simulink model "zad2_modell"  (R2023a)
settings: Solver=ode45  StartTime=0.0  StopTime=Tsim  RelTol=1e-3  EnableMultiTasking=on
values from neighbouring files (symbols this model uses):
  beta = Ks*Kg*Km/(Jl*Jh*Rm)    (= 26833.3333333)    [zad2_b.m]
  Jh = 0.0021    [zad2_a.m]    (also in zad2_b.m)
  Jl = 0.0059    [zad2_a.m]    (also in zad2_b.m)
  K = acker(A_, B_, p)    [zad2_b.m]
  Kg = 70    [zad2_a.m]    (also in zad2_b.m)
  Km = 0.00767    [zad2_a.m]    (also in zad2_b.m)
  konst = m*g*h/Jl    (= -39.9050847458)    [zad2_b.m]
  Ks = 1.61    [zad2_a.m]    (also in zad2_b.m)
  Rm = 2.6    [zad2_a.m]    (also in zad2_b.m)
settings Model: Creator=Guzda  LastModifiedBy=Enio
settings SolverCC: AlgebraicLoopSolver=TrustRegion
settings DataIOCC: LimitDataPoints=on  SaveFormat=Array  SignalLoggingSaveFormat=ModelDataLogs  ReturnWorkspaceOutputs=off
settings OptimizationCC: LifeSpan=inf
settings DebuggingCC: UnderspecifiedInitializationDetection=Classic  MergeDetectMultiDrivingBlocksExec=none  MultiTaskDSMMsg=warning  MultiTaskCondExecSysMsg=none  UnconnectedInputMsg=warning  UnconnectedOutputMsg=warning  UnconnectedLineMsg=warning  StateNameClashWarn=warning  SFUnexpectedBacktrackingDiag=warning  SFNoUnconditionalDefaultTransitionDiag=warning  SFExecutionAtInitializationDiag=none  ArithmeticOperatorsInVariantConditions=warning
settings HardwareCC: ProdBitPerPointer=32  ProdBitPerSizeT=32  ProdBitPerPtrDiffT=32  ProdLargestAtomicFloat=None  ProdIntDivRoundTo=Undefined  ProdEndianess=Unspecified  ProdWordSize=32  ProdHWDeviceType=32-bit Generic
settings ModelReferenceCC: EnableRefExpFcnMdlSchedulingChecks=on  PropagateSignalLabelsOutOfModel=off
settings SFSimCC: SimUseLocalCustomCode=off  CustomCodeUndefinedFunction=UseInterfaceOnly
settings RTWCC: RTWUseLocalCustomCode=off
settings CodeAppCC: StateflowObjectComments=on
settings GRTTargetCC: TargetLangStandard=C89/C90 (ANSI)
settings ConfigComp: CovMetricSettings=dw  CovSaveCumulativeToWorkspaceVar=on  CovSaveSingleToWorkspaceVar=on  CovExternalEMLEnable=off

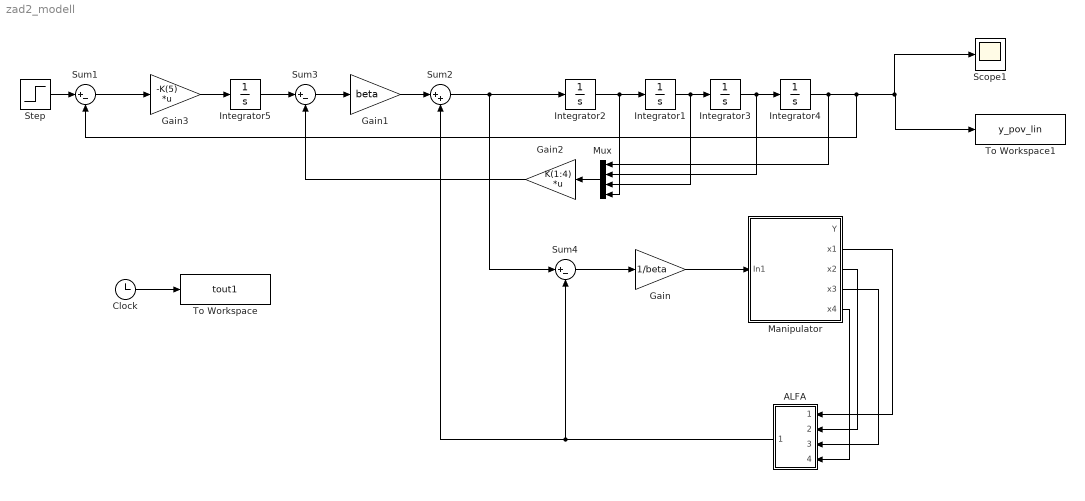
== system zad2_modell ==
  ALFA : Subsystem
  Clock : Clock
  Gain : Gain  Gain=1/beta
  Gain1 : Gain  Gain=beta
  Gain2 : Gain  Gain=K(1:4)  Multiplication=Matrix(K*u)
  Gain3 : Gain  Gain=-K(5)  Multiplication=Matrix(K*u)
  Integrator{1..5} (5 alike) : Integrator
  Manipulator : Subsystem
  Mux : Mux
  Scope1 : Scope
  Step : Step  Time=0  After=u  SampleTime=0
  Sum1 : Sum  Inputs=|+-
  Sum2 : Sum  Inputs=|++
  Sum3 : Sum  Inputs=|+-
  Sum4 : Sum  Inputs=|+-
  To Workspace : ToWorkspace  VariableName=tout1  SampleTime=-1
  To Workspace1 : ToWorkspace  VariableName=y_pov_lin  SampleTime=-1
  wires:
  Clock/1 -> To Workspace/1
  Manipulator/4(x3) -> ALFA/3(In3)
  Manipulator/5(x4) -> ALFA/4(In4)
  Manipulator/3(x2) -> ALFA/2(In2)
  Gain/1 -> Manipulator/1(In1)
  Integrator2/1 -> Mux/4, Integrator1/1
  Integrator1/1 -> Mux/3, Integrator3/1
  Integrator3/1 -> Mux/2, Integrator4/1
  Integrator4/1 -> Mux/1, Sum1/2, To Workspace1/1, Scope1/1
  ALFA/1(Out1) -> Sum4/2, Sum2/2
  Sum2/1 -> Sum4/1, Integrator2/1
  Gain1/1 -> Sum2/1
  Sum3/1 -> Gain1/1
  Mux/1 -> Gain2/1
  Gain2/1 -> Sum3/2
  Integrator5/1 -> Sum3/1
  Gain3/1 -> Integrator5/1
  Sum1/1 -> Gain3/1
  Step/1 -> Sum1/1
  Sum4/1 -> Gain/1
  Manipulator/2(x1) -> ALFA/1(In1)

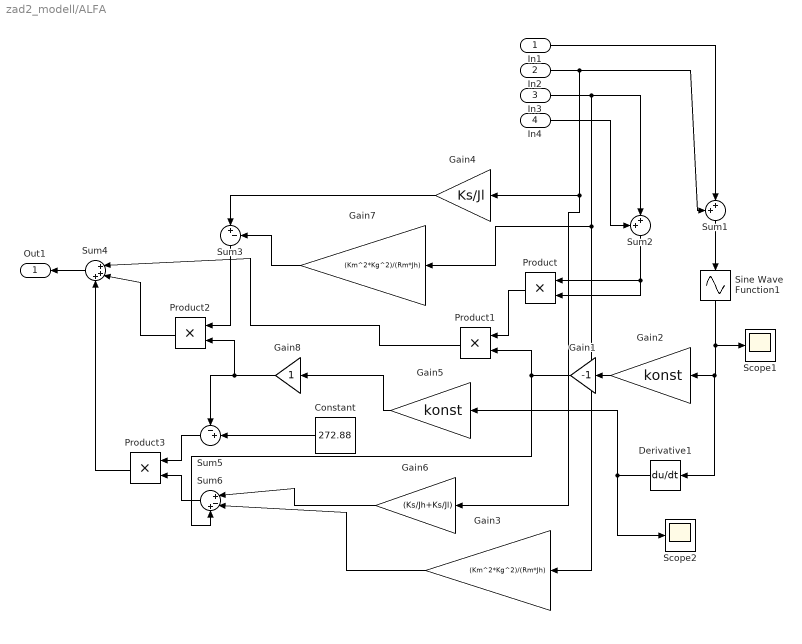
== system zad2_modell/ALFA ==
  In1 : Inport
  In2 : Inport  Port=2
  In3 : Inport  Port=3
  In4 : Inport  Port=4
  Constant : Constant  Value=272.88
  Derivative1 : Derivative
  Gain1 : Gain  Gain=-1
  Gain2 : Gain  Gain=konst
  Gain3 : Gain  Gain=(Km^2*Kg^2)/(Rm*Jh)
  Gain4 : Gain  Gain=Ks/Jl
  Gain5 : Gain  Gain=konst
  Gain6 : Gain  Gain=(Ks/Jh+Ks/Jl)
  Gain7 : Gain  Gain=(Km^2*Kg^2)/(Rm*Jh)
  Gain8 : Gain
  Product{,1..3} (4 alike) : Product
  Scope1 : Scope
  Scope2 : Scope
  Sine Wave Function1 : Sin  TimeSource=Use external signal  SampleTime=0
  Sum1 : Sum  Inputs=++|
  Sum2 : Sum  Inputs=++|
  Sum3 : Sum  Inputs=|+-
  Sum4 : Sum  Inputs=|+++
  Sum5 : Sum  Inputs=-+|
  Sum6 : Sum  Inputs=|+-+
  Out1 : Outport
  wires:
  Sine Wave Function1/1 -> Scope1/1, Derivative1/1, Gain2/1
  Product/1 -> Product1/1
  Gain8/1 -> Sum5/1, Product2/2
  Constant/1 -> Sum5/2
  Sum3/1 -> Product2/1
  Gain4/1 -> Sum3/1
  Gain1/1 -> Sum6/3, Product1/2
  Gain7/1 -> Sum3/2
  Product2/1 -> Sum4/2
  Product1/1 -> Sum4/1
  Gain2/1 -> Gain1/1
  In4/1 -> Sum2/1
  In2/1 -> Gain6/1, Gain4/1, Sum1/1
  In1/1 -> Sum1/2
  In3/1 -> Gain3/1, Gain7/1, Sum2/2
  Sum1/1 -> Sine Wave Function1/1
  Sum2/1 -> Product/2, Product/1
  Product3/1 -> Sum4/3
  Sum6/1 -> Product3/2
  Gain6/1 -> Sum6/1
  Gain3/1 -> Sum6/2
  Sum5/1 -> Product3/1
  Sum4/1 -> Out1/1
  Gain5/1 -> Gain8/1
  Derivative1/1 -> Scope2/1, Gain5/1

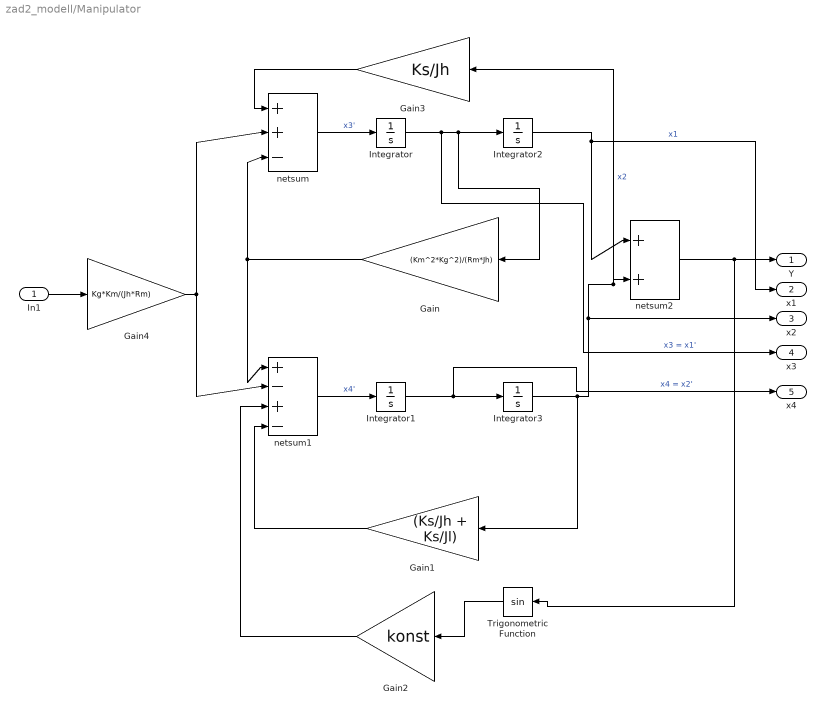
== system zad2_modell/Manipulator ==
  In1 : Inport
  Gain : Gain  Gain=(Km^2*Kg^2)/(Rm*Jh)
  Gain1 : Gain  Gain=(Ks/Jh + Ks/Jl)
  Gain2 : Gain  Gain=konst
  Gain3 : Gain  Gain=Ks/Jh
  Gain4 : Gain  Gain=Kg*Km/(Jh*Rm)
  Integrator{,1..3} (4 alike) : Integrator
  Trigonometric Function : Trigonometry
  netsum : Sum  Inputs=|++-  InputSameDT=on  SaturateOnIntegerOverflow=on  OutDataTypeStr=Inherit: Same as first input
  netsum1 : Sum  Inputs=|+-+-  InputSameDT=on  SaturateOnIntegerOverflow=on  OutDataTypeStr=Inherit: Same as first input
  netsum2 : Sum  Inputs=|++  InputSameDT=on  SaturateOnIntegerOverflow=on  OutDataTypeStr=Inherit: Same as first input
  Y : Outport
  x1 : Outport  Port=2
  x2 : Outport  Port=3
  x3 : Outport  Port=4
  x4 : Outport  Port=5
  wires:
  Integrator1/1 -> Integrator3/1, x4/1  "x4 = x2'"
  netsum1/1 -> Integrator1/1  "x4'"
  Integrator2/1 -> netsum2/1, x1/1  "x1"
  netsum2/1 -> Trigonometric Function/1, Y/1
  Gain4/1 -> netsum1/2, netsum/2
  Gain1/1 -> netsum1/4
  netsum/1 -> Integrator/1  "x3'"
  Integrator3/1 -> Gain1/1, Gain3/1, netsum2/2, x2/1  "x2"
  Gain/1 -> netsum/3, netsum1/1
  Integrator/1 -> Integrator2/1, Gain/1, x3/1  "x3 = x1'"
  Gain3/1 -> netsum/1
  Gain2/1 -> netsum1/3
  In1/1 -> Gain4/1
  Trigonometric Function/1 -> Gain2/1
